simulink model "WDGBrakingLogic"  (R2024a)
settings: configuration reference "csMultiInstance" (kept outside this file)
undefined symbols (not defined in the file or in its folder): Default_decel, FB_decel, StopTime_Max, StopTime_Min, stopVelThreshold, Ts, TTC_Max, TTC_Min, Velocity_Max, Velocity_Min
Description:
  | Software unit for WDG braking logic
settings Model: DataDictionary=DD_WDGBrakingLogic.sldd  EnableAccessToBaseWorkspace=off  Creator=The MathWorks, Inc.  LastModifiedBy=The MathWorks, Inc.
settings ConfigSetRef: SourceName=csMultiInstance

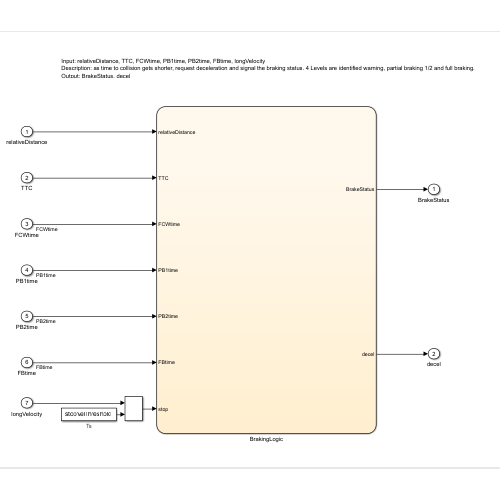
[thumbnail: Simulink's stored preview of the top-level diagram]
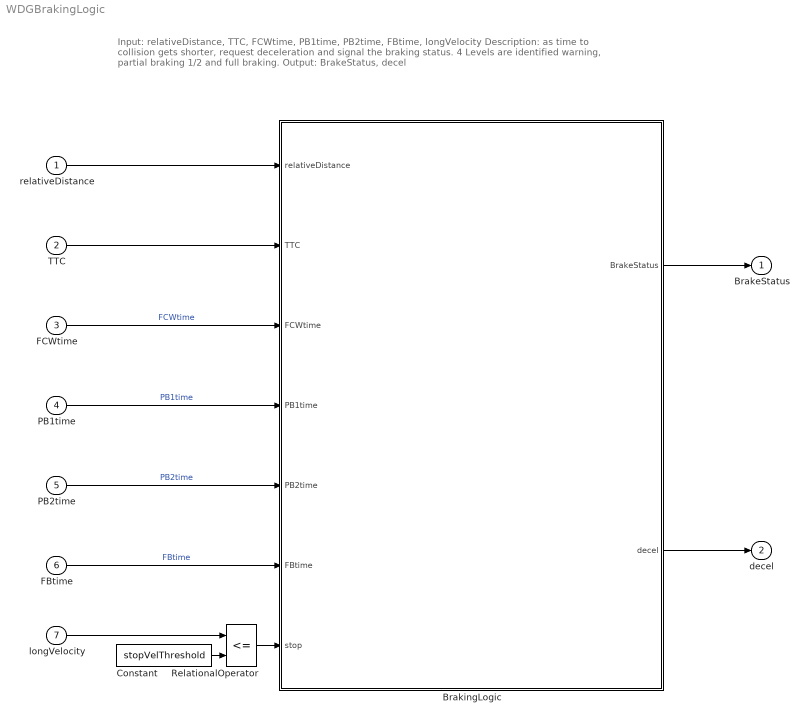
== system WDGBrakingLogic ==
  note: Input: relativeDistance, TTC, FCWtime, PB1time, PB2time, FBtime, longVelocity
      | Description: as time to collision gets shorter, request deceleration and signal the braking status. 4 Levels are identified warning, partial braking 1/2 and full braking.
      | Output: BrakeStatus, decel
  relativeDistance : Inport  OutDataTypeStr=Distance_DType  Unit=m  PortDimensions=Distance_Dimensions  SampleTime=Ts
  TTC : Inport  Port=2  OutMin=TTC_Min  OutMax=TTC_Max  OutDataTypeStr=TTC_DType  Unit=s  PortDimensions=TTC_Dimensions  SampleTime=Ts
  FCWtime : Inport  Port=3  OutMin=StopTime_Min  OutMax=StopTime_Max  OutDataTypeStr=StopTime_DType  Unit=s  PortDimensions=StopTime_Dimensions  SampleTime=Ts
  PB1time : Inport  Port=4  OutMin=StopTime_Min  OutMax=StopTime_Max  OutDataTypeStr=StopTime_DType  Unit=s  PortDimensions=StopTime_Dimensions  SampleTime=Ts
  PB2time : Inport  Port=5  OutMin=StopTime_Min  OutMax=StopTime_Max  OutDataTypeStr=StopTime_DType  Unit=s  PortDimensions=StopTime_Dimensions  SampleTime=Ts
  FBtime : Inport  Port=6  OutMin=StopTime_Min  OutMax=StopTime_Max  OutDataTypeStr=StopTime_DType  Unit=s  PortDimensions=StopTime_Dimensions  SampleTime=Ts
  longVelocity : Inport  Port=7  OutMin=Velocity_Min  OutMax=Velocity_Max  OutDataTypeStr=Velocity_DType  Unit=m/s  PortDimensions=Velocity_Dimensions  SampleTime=Ts
  BrakingLogic : Stateflow chart  TreatAsAtomicUnit=on
  Constant : Constant  Value=stopVelThreshold  SampleTime=Ts
      settings: AttributesFormatString=%<SampleTime>
  RelationalOperator : RelationalOperator  Operator=<=  RndMeth=Simplest  InputSameDT=off
  BrakeStatus : Outport  OutDataTypeStr=Enum: BrStatus  PortDimensions=BrStatus_Dimensions  SampleTime=Ts  VectorParamsAs1DForOutWhenUnconnected=off
  decel : Outport  Port=2  OutMin=Default_decel  OutMax=FB_decel  OutDataTypeStr=Acceleration_DType  Unit=m/s^2  PortDimensions=Acceleration_Dimensions  SampleTime=Ts  VectorParamsAs1DForOutWhenUnconnected=off
  wires:
  BrakingLogic/2(decel) -> decel/1
  BrakingLogic/1(BrakeStatus) -> BrakeStatus/1
  TTC/1 -> BrakingLogic/2(TTC)
  PB1time/1 -> BrakingLogic/4(PB1time)  "PB1time"
  relativeDistance/1 -> BrakingLogic/1(relativeDistance)
  FCWtime/1 -> BrakingLogic/3(FCWtime)  "FCWtime"
  PB2time/1 -> BrakingLogic/5(PB2time)  "PB2time"
  FBtime/1 -> BrakingLogic/6(FBtime)  "FBtime"
  longVelocity/1 -> RelationalOperator/1
  RelationalOperator/1 -> BrakingLogic/7(stop)
  Constant/1 -> RelationalOperator/2

== stateflow chart WDGBrakingLogic/BrakingLogic ==
  state Default
    entry:
    BrakeStatus = BrStatus.NoBrake;
    decel = Default_decel;
  state FCW
    entry:
    BrakeStatus = BrStatus.NoBrake;
    decel = Default_decel;
  state Partial_Braking1
    entry:
    BrakeStatus = BrStatus.PB1Brake;
    decel = PB1_decel;
  state Partial_Braking2
    entry:
    BrakeStatus =BrStatus.PB2Brake;
    decel = PB2_decel;
  state Full_Braking
    entry:
    BrakeStatus = BrStatus.FBrake;
    decel = FB_decel;
  (default) -> Default
  Default -> (junction 114) [order 2]
  (junction 114) -> Full_Braking : [relativeDistance < default_spacing]
  (junction 95) -> Default
  Full_Braking -> (junction 95) : [stop && TTC>double(0) && relativeDistance > default_spacing ]
  (junction 101) -> Default
  (junction 103) -> (junction 101) : [stop]
  (junction 97) -> Default
  (junction 99) -> (junction 97) : [stop]
  Default -> FCW [order 1] : [(abs(TTC)<FCWtime) && TTC<double(0)]
  FCW -> Default [order 2] : [abs(TTC)>=TimeFactor*FCWtime]
  FCW -> Partial_Braking1 [order 1] : [(abs(TTC) < PB1time) && TTC<double(0)]
  Partial_Braking1 -> (junction 99) [order 2]
  Partial_Braking1 -> Partial_Braking2 [order 1] : [(abs(TTC) < PB2time) && TTC<double(0)]
  Partial_Braking2 -> (junction 103) [order 2]
  Partial_Braking2 -> Full_Braking [order 1] : [(abs(TTC) < FBtime) && TTC<double(0)]
  data: relativeDistance input; TTC input; FCWtime input; PB1time input; PB2time input; FBtime input; BrakeStatus output; decel output; stop input boolean; FB_decel constant double =FB_decel; PB2_decel constant double =PB2_decel; Default_decel constant double =Default_decel; TimeFactor constant double =TimeFactor; PB1_decel constant double =PB1_decel; default_spacing constant double =default_spacing
